simulink library "constXY_ZTVarADCP_cl"  (R2018b)
settings: Solver=VariableStepAuto  StartTime=0.0  StopTime=10.0  RelTol=1e-3
undefined symbols (not defined in the file): env
libraries: variableFlowProfileCalculation_ul x1
settings Model: Creator=jcreed2  LastModifiedBy=jcreed2

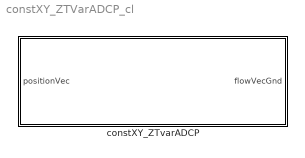
== system constXY_ZTVarADCP_cl ==
  constXY_ZTvarADCP : Subsystem

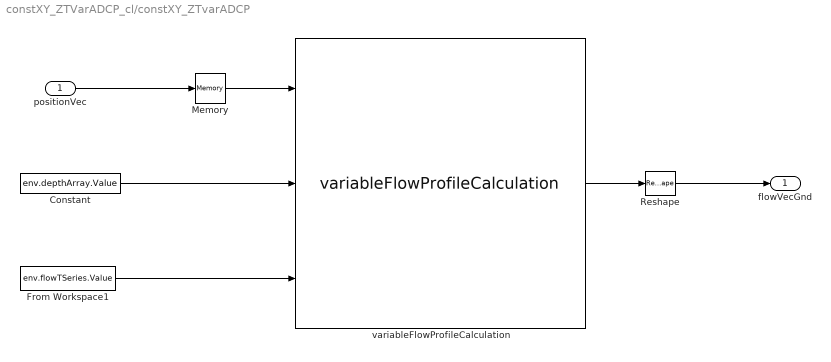
== system constXY_ZTVarADCP_cl/constXY_ZTvarADCP ==
  "positionVec " : Inport
  Constant : Constant  Value=env.depthArray.Value
  From Workspace1 : FromWorkspace  VariableName=env.flowTSeries.Value  SampleTime=0
  Memory : Memory
  Reshape : Reshape  OutputDimensionality=Column vector (2-D)
  variableFlowProfileCalculation : variableFlowProfileCalculation_ul/variableFlowProfileCalculation  SystemSampleTime=-1
  flowVecGnd : Outport
  wires:
  Constant/1 -> variableFlowProfileCalculation/2
  variableFlowProfileCalculation/1 -> Reshape/1
  "positionVec "/1 -> Memory/1
  From Workspace1/1 -> variableFlowProfileCalculation/3
  Reshape/1 -> flowVecGnd/1
  Memory/1 -> variableFlowProfileCalculation/1
